simulink library "aero"  (R2022b)
settings: Solver=VariableStepAuto  StartTime=0.0  StopTime=10.0  RelTol=1e-3
values from neighbouring files (symbols this model uses):
  alpha_da = (-3:3:12)'    [load_mdl_data.m]
  alpha_de = (-2:2:14)'    [load_mdl_data.m]
  alpha_dr = (-3:3:12)'    [load_mdl_data.m]
  alpha_dyn = [4,6,8]    [load_mdl_data.m]
  alpha_lat = (-2:2:8)'    [load_mdl_data.m]
  alpha_lon = (-2:2:18)'    [load_mdl_data.m]
  beta_lat = -6:3:6    [load_mdl_data.m]
  CD_base = data_base(:,2)    [load_mdl_data.m]
  CD_beta = [data_beta_n6(:,2)-interp1(alpha_lon,CD_base, alpha_lat),      data_beta_n3(:,2)-interp1(alpha_lon,CD_base, alpha_lat),      zeros(size(data_beta_n3(:,2))),      data_beta_p3(:,2)-interp1(alpha_lon,CD_base, alpha_lat),      data_beta_p6(:,2)-interp1(alpha_lon,CD_base, alpha_lat)]    [load_mdl_data.m]
  CD_da = [data_da_n15(:,2)-interp1(alpha_lon,CD_base, alpha_da,'linear','extrap'),      zeros(size(data_da_n15(:,2))),      data_da_p15(:,2)-interp1(alpha_lon,CD_base, alpha_da,'linear','extrap')]/15    [load_mdl_data.m]
  CD_de = [(data_de_n15(:,2)-interp1(alpha_lon,CD_base, alpha_de,'linear','extrap'))/-15,      (data_de_p15(:,2)-data_de_n15(:,2))/30,      (data_de_p15(:,2)-interp1(alpha_lon,CD_base, alpha_de,'linear','extrap'))/15]    [load_mdl_data.m]
  CD_dr = [data_dr_n15(:,2)-interp1(alpha_lon,CD_base, alpha_dr,'linear','extrap'),      zeros(size(data_dr_n15(:,2))),      data_dr_p15(:,2)-interp1(alpha_lon,CD_base, alpha_dr,'linear','extrap')]/15    [load_mdl_data.m]
  CL_base = data_base(:,1)    [load_mdl_data.m]
  Cl_base = data_base(:,5)    [load_mdl_data.m]
  CL_beta = [data_beta_n6(:,1)-interp1(alpha_lon,CL_base, alpha_lat),      data_beta_n3(:,1)-interp1(alpha_lon,CL_base, alpha_lat),      zeros(size(data_beta_n3(:,1))),      data_beta_p3(:,1)-interp1(alpha_lon,CL_base, alpha_lat),      data_beta_p6(:,1)-interp1(alpha_lon,CL_base, alpha_lat)]    [load_mdl_data.m]
  Cl_beta = [data_beta_n6(:,5)-interp1(alpha_lon,Cl_base, alpha_lat),      data_beta_n3(:,5)-interp1(alpha_lon,Cl_base, alpha_lat),      zeros(size(data_beta_n3(:,5))),      data_beta_p3(:,5)-interp1(alpha_lon,Cl_base, alpha_lat),      data_beta_p6(:,5)-interp1(alpha_lon,Cl_base, alpha_lat)]    [load_mdl_data.m]
  CL_da = [data_da_n15(:,1)-interp1(alpha_lon,CL_base, alpha_da,'linear','extrap'),      zeros(size(data_da_n15(:,1))),      data_da_p15(:,1)-interp1(alpha_lon,CL_base, alpha_da,'linear','extrap')]/15    [load_mdl_data.m]
  Cl_da = [(data_da_n15(:,5)-interp1(alpha_lon,Cl_base, alpha_da,'linear','extrap'))/-15,      (data_da_p15(:,5)-data_da_n15(:,5))/30,      (data_da_p15(:,5)-interp1(alpha_lon,Cl_base, alpha_da,'linear','extrap'))/15]    [load_mdl_data.m]
  CL_de = [(data_de_n15(:,1)-interp1(alpha_lon,CL_base, alpha_de,'linear','extrap'))/-15,      (data_de_p15(:,1)-data_de_n15(:,1))/30,      (data_de_p15(:,1)-interp1(alpha_lon,CL_base, alpha_de,'linear','extrap'))/15]    [load_mdl_data.m]
  CL_dr = [data_dr_n15(:,1)-interp1(alpha_lon,CL_base, alpha_dr,'linear','extrap'),      zeros(size(data_dr_n15(:,1))),      data_dr_p15(:,1)-interp1(alpha_lon,CL_base, alpha_dr,'linear','extrap')]/15    [load_mdl_data.m]
  Cl_dr = [(data_dr_n15(:,5)-interp1(alpha_lon,Cl_base, alpha_dr,'linear','extrap'))/-15,      (data_dr_p15(:,5)-data_dr_n15(:,5))/30,      (data_dr_p15(:,5)-interp1(alpha_lon,Cl_base, alpha_dr,'linear','extrap'))/15]    [load_mdl_data.m]
  Clp = [-0.7,  -0.66, -0.58]    [load_mdl_data.m]
  CLq = [71,    60,    55]    [load_mdl_data.m]
  Clr = [0.39,   0.45,  0.52]    [load_mdl_data.m]
  Cm_base = data_base(:,4)    [load_mdl_data.m]
  Cm_beta = [data_beta_n6(:,4)-interp1(alpha_lon,Cm_base, alpha_lat),      data_beta_n3(:,4)-interp1(alpha_lon,Cm_base, alpha_lat),      zeros(size(data_beta_n3(:,4))),      data_beta_p3(:,4)-interp1(alpha_lon,Cm_base, alpha_lat),      data_beta_p6(:,4)-interp1(alpha_lon,Cm_base, alpha_lat)]    [load_mdl_data.m]
  Cm_da = [data_da_n15(:,4)-interp1(alpha_lon,Cm_base, alpha_da,'linear','extrap'),      zeros(size(data_da_n15(:,4))),      data_da_p15(:,4)-interp1(alpha_lon,Cm_base, alpha_da,'linear','extrap')]/15    [load_mdl_data.m]
  Cm_de = [(data_de_n15(:,4)-interp1(alpha_lon,Cm_base, alpha_de,'linear','extrap'))/-15,      (data_de_p15(:,4)-data_de_n15(:,4))/30,      (data_de_p15(:,4)-interp1(alpha_lon,Cm_base, alpha_de,'linear','extrap'))/15]    [load_mdl_data.m]
  Cm_dr = [data_dr_n15(:,4)-interp1(alpha_lon,Cm_base, alpha_dr,'linear','extrap'),      zeros(size(data_dr_n15(:,4))),      data_dr_p15(:,4)-interp1(alpha_lon,Cm_base, alpha_dr,'linear','extrap')]/15    [load_mdl_data.m]
  Cmq = [-54,  -55,   -55]    [load_mdl_data.m]
  Cn_base = data_base(:,6)    [load_mdl_data.m]
  Cn_beta = [data_beta_n6(:,6)-interp1(alpha_lon,Cn_base, alpha_lat),      data_beta_n3(:,6)-interp1(alpha_lon,Cn_base, alpha_lat),      zeros(size(data_beta_n3(:,6))),      data_beta_p3(:,6)-interp1(alpha_lon,Cn_base, alpha_lat),      data_beta_p6(:,6)-interp1(alpha_lon,Cn_base, alpha_lat)]    [load_mdl_data.m]
  Cn_da = [(data_da_n15(:,6)-interp1(alpha_lon,Cn_base, alpha_da,'linear','extrap'))/-15,      (data_da_p15(:,6)-data_da_n15(:,6))/30,      (data_da_p15(:,6)-interp1(alpha_lon,Cn_base, alpha_da,'linear','extrap'))/15]    [load_mdl_data.m]
  Cn_dr = [(data_dr_n15(:,6)-interp1(alpha_lon,Cn_base, alpha_dr,'linear','extrap'))/-15,      (data_dr_p15(:,6)-data_dr_n15(:,6))/30,      (data_dr_p15(:,6)-interp1(alpha_lon,Cn_base, alpha_dr,'linear','extrap'))/15]    [load_mdl_data.m]
  Cnp = [-0.07, -0.08, -0.09]    [load_mdl_data.m]
  Cnr = [-0.12, -0.13, -0.14]    [load_mdl_data.m]
  Cs_base = data_base(:,3)    [load_mdl_data.m]
  Cs_beta = [data_beta_n6(:,3)-interp1(alpha_lon,Cs_base, alpha_lat),      data_beta_n3(:,3)-interp1(alpha_lon,Cs_base, alpha_lat),      zeros(size(data_beta_n3(:,3))),      data_beta_p3(:,3)-interp1(alpha_lon,Cs_base, alpha_lat),      data_beta_p6(:,3)-interp1(alpha_lon,Cs_base, alpha_lat)]    [load_mdl_data.m]
  Cs_da = [(data_da_n15(:,3)-interp1(alpha_lon,Cs_base, alpha_da,'linear','extrap'))/-15,      (data_da_p15(:,3)-data_da_n15(:,3))/30,      (data_da_p15(:,3)-interp1(alpha_lon,Cs_base, alpha_da,'linear','extrap'))/15]    [load_mdl_data.m]
  Cs_dr = [(data_dr_n15(:,3)-interp1(alpha_lon,Cs_base, alpha_dr,'linear','extrap'))/-15,      (data_dr_p15(:,3)-data_dr_n15(:,3))/30,      (data_dr_p15(:,3)-interp1(alpha_lon,Cs_base, alpha_dr,'linear','extrap'))/15]    [load_mdl_data.m]
  da_bp = [-15 0 15]    [load_mdl_data.m]
  de_bp = [-15 0 15]    [load_mdl_data.m]
  dr_bp = [-15 0 15]    [load_mdl_data.m]
  RefLen = 0.18    [load_mdl_data.m]
  RefSpan = 3.2    [load_mdl_data.m]
libraries: simulink_extras x5
settings Model: Creator=matt  LastModifiedBy=matt

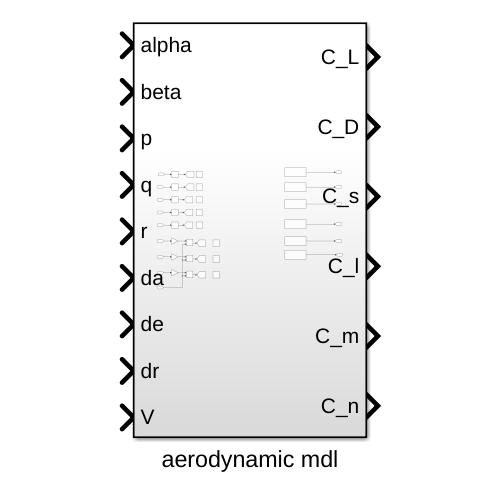
[thumbnail: Simulink's stored preview of the top-level diagram]
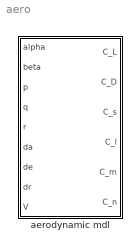
== system aero ==
  aerodynamic mdl : Subsystem

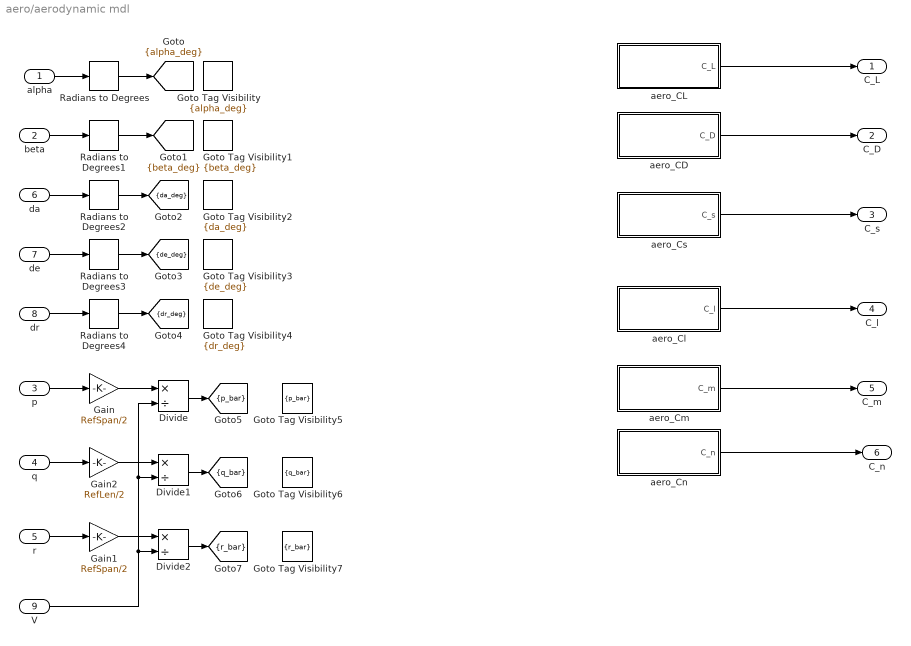
== system aero/aerodynamic mdl ==
  alpha : Inport
  beta : Inport  Port=2
  p : Inport  Port=3
  q : Inport  Port=4
  r : Inport  Port=5
  da : Inport  Port=6
  de : Inport  Port=7
  dr : Inport  Port=8
  V : Inport  Port=9
  Divide : Product  Inputs=*/
  Divide1 : Product  Inputs=*/
  Divide2 : Product  Inputs=*/
  Gain : Gain  Gain=RefSpan/2
  Gain1 : Gain  Gain=RefSpan/2
  Gain2 : Gain  Gain=RefLen/2
  Goto Tag Visibility : GotoTagVisibility  GotoTag=alpha_deg
  Goto Tag Visibility1 : GotoTagVisibility  GotoTag=beta_deg
  Goto Tag Visibility2 : GotoTagVisibility  GotoTag=da_deg
  Goto Tag Visibility3 : GotoTagVisibility  GotoTag=de_deg
  Goto Tag Visibility4 : GotoTagVisibility  GotoTag=dr_deg
  Goto Tag Visibility5 : GotoTagVisibility  GotoTag=p_bar
  Goto Tag Visibility6 : GotoTagVisibility  GotoTag=q_bar
  Goto Tag Visibility7 : GotoTagVisibility  GotoTag=r_bar
  Radians to Degrees{,1..4} (5 alike) : simulink_extras/Transformations/Radians to Degrees
  aero_CD : Subsystem
  aero_CL : Subsystem
  aero_Cl : Subsystem
  aero_Cm : Subsystem
  aero_Cn : Subsystem
  aero_Cs : Subsystem
  C_L : Outport
  C_D : Outport  Port=2
  C_s : Outport  Port=3
  C_l : Outport  Port=4
  C_m : Outport  Port=5
  C_n : Outport  Port=6
  tag scope: alpha_deg=scoped, beta_deg=scoped, da_deg=scoped, de_deg=scoped, dr_deg=scoped, p_bar=scoped, q_bar=scoped, r_bar=scoped
  wires:
  alpha/1 -> Radians to Degrees/1
  beta/1 -> Radians to Degrees1/1
  Radians to Degrees/1 -> [alpha_deg]
  Radians to Degrees1/1 -> [beta_deg]
  dr/1 -> Radians to Degrees4/1
  de/1 -> Radians to Degrees3/1
  da/1 -> Radians to Degrees2/1
  Radians to Degrees2/1 -> [da_deg]
  Radians to Degrees3/1 -> [de_deg]
  Radians to Degrees4/1 -> [dr_deg]
  p/1 -> Gain/1
  r/1 -> Gain1/1
  q/1 -> Gain2/1
  Gain/1 -> Divide/1
  V/1 -> Divide2/2, Divide1/2, Divide/2
  Divide/1 -> [p_bar]
  Divide1/1 -> [q_bar]
  Gain2/1 -> Divide1/1
  Divide2/1 -> [r_bar]
  Gain1/1 -> Divide2/1
  aero_CL/1(C_L) -> C_L/1
  aero_Cm/1(C_m) -> C_m/1
  aero_CD/1(C_D) -> C_D/1
  aero_Cs/1(C_s) -> C_s/1
  aero_Cl/1(C_l) -> C_l/1
  aero_Cn/1(C_n) -> C_n/1

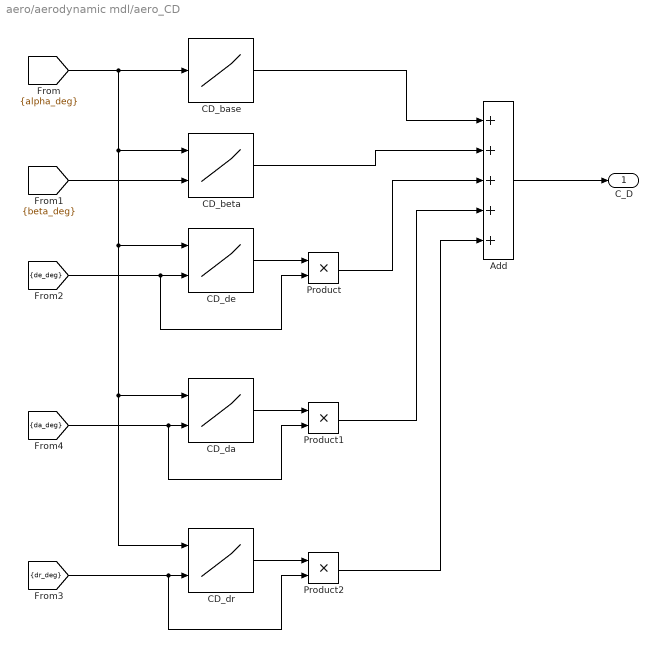
== system aero/aerodynamic mdl/aero_CD ==
  Add : Sum  Inputs=+++++
  CD_base : Lookup_n-D  NumberOfTableDimensions=1  BreakpointsForDimension1=alpha_lon  BeginIndexSearchUsingPreviousIndexResult=on  Table=CD_base  InternalRulePriority=Speed  RndMeth=Simplest
  CD_beta : Lookup_n-D  BreakpointsForDimension1=alpha_lat  BreakpointsForDimension2=beta_lat  BeginIndexSearchUsingPreviousIndexResult=on  Table=CD_beta  InternalRulePriority=Speed  RndMeth=Simplest
      settings: InputPortMap=u0,u1
  CD_da : Lookup_n-D  BreakpointsForDimension1=alpha_da  BreakpointsForDimension2=da_bp  BeginIndexSearchUsingPreviousIndexResult=on  Table=CD_da  ExtrapMethod=Clip  InternalRulePriority=Speed  RndMeth=Simplest
      settings: InputPortMap=u0,u1
  CD_de : Lookup_n-D  BreakpointsForDimension1=alpha_de  BreakpointsForDimension2=de_bp  BeginIndexSearchUsingPreviousIndexResult=on  Table=CD_de  ExtrapMethod=Clip  InternalRulePriority=Speed  RndMeth=Simplest
      settings: InputPortMap=u0,u1
  CD_dr : Lookup_n-D  BreakpointsForDimension1=alpha_dr  BreakpointsForDimension2=dr_bp  BeginIndexSearchUsingPreviousIndexResult=on  Table=CD_dr  ExtrapMethod=Clip  InternalRulePriority=Speed  RndMeth=Simplest
      settings: InputPortMap=u0,u1
  Product : Product
  Product1 : Product
  Product2 : Product
  C_D : Outport
  wires:
  Product2/1 -> Add/5
  [dr_deg] -> CD_dr/2, Product2/2
  CD_dr/1 -> Product2/1
  [alpha_deg] -> CD_base/1, CD_beta/1, CD_de/1, CD_da/1, CD_dr/1
  Product1/1 -> Add/4
  [da_deg] -> CD_da/2, Product1/2
  CD_da/1 -> Product1/1
  Product/1 -> Add/3
  [de_deg] -> CD_de/2, Product/2
  CD_de/1 -> Product/1
  [beta_deg] -> CD_beta/2
  CD_beta/1 -> Add/2
  CD_base/1 -> Add/1
  Add/1 -> C_D/1

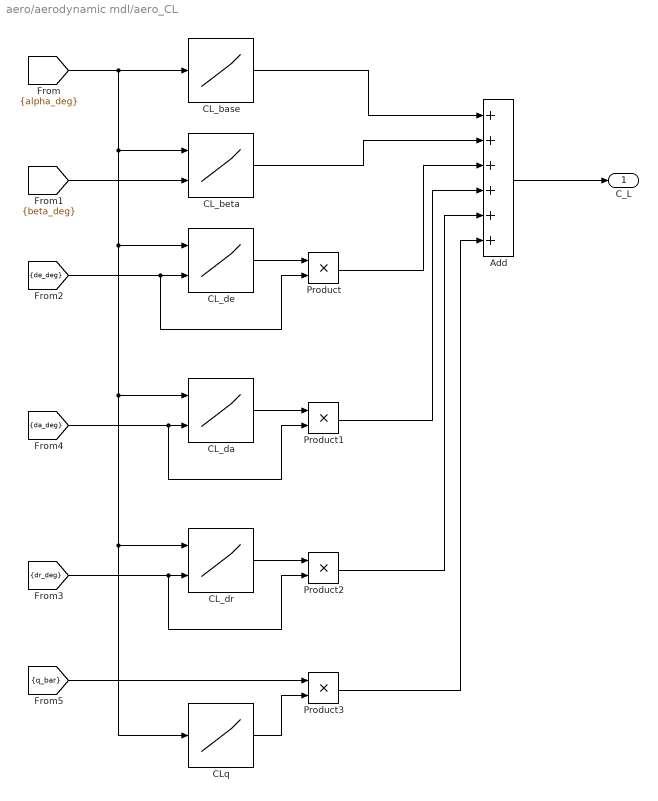
== system aero/aerodynamic mdl/aero_CL ==
  Add : Sum  Inputs=++++++
  CL_base : Lookup_n-D  NumberOfTableDimensions=1  BreakpointsForDimension1=alpha_lon  BeginIndexSearchUsingPreviousIndexResult=on  Table=CL_base  InternalRulePriority=Speed  RndMeth=Simplest
  CL_beta : Lookup_n-D  BreakpointsForDimension1=alpha_lat  BreakpointsForDimension2=beta_lat  BeginIndexSearchUsingPreviousIndexResult=on  Table=CL_beta  InternalRulePriority=Speed  RndMeth=Simplest
      settings: InputPortMap=u0,u1
  CL_da : Lookup_n-D  BreakpointsForDimension1=alpha_da  BreakpointsForDimension2=da_bp  BeginIndexSearchUsingPreviousIndexResult=on  Table=CL_da  ExtrapMethod=Clip  InternalRulePriority=Speed  RndMeth=Simplest
      settings: InputPortMap=u0,u1
  CL_de : Lookup_n-D  BreakpointsForDimension1=alpha_de  BreakpointsForDimension2=de_bp  BeginIndexSearchUsingPreviousIndexResult=on  Table=CL_de  ExtrapMethod=Clip  InternalRulePriority=Speed  RndMeth=Simplest
      settings: InputPortMap=u0,u1
  CL_dr : Lookup_n-D  BreakpointsForDimension1=alpha_dr  BreakpointsForDimension2=dr_bp  BeginIndexSearchUsingPreviousIndexResult=on  Table=CL_dr  ExtrapMethod=Clip  InternalRulePriority=Speed  RndMeth=Simplest
      settings: InputPortMap=u0,u1
  CLq : Lookup_n-D  NumberOfTableDimensions=1  BreakpointsForDimension1=alpha_dyn  BeginIndexSearchUsingPreviousIndexResult=on  Table=CLq  ExtrapMethod=Clip  UseLastTableValue=on  InternalRulePriority=Speed  RndMeth=Simplest
  Product{,1..3} (4 alike) : Product
  C_L : Outport
  wires:
  Add/1 -> C_L/1
  CL_base/1 -> Add/1
  CL_beta/1 -> Add/2
  [beta_deg] -> CL_beta/2
  CL_de/1 -> Product/1
  [de_deg] -> Product/2, CL_de/2
  Product/1 -> Add/3
  CL_da/1 -> Product1/1
  [da_deg] -> Product1/2, CL_da/2
  Product1/1 -> Add/4
  [alpha_deg] -> CLq/1, CL_dr/1, CL_da/1, CL_de/1, CL_beta/1, CL_base/1
  CL_dr/1 -> Product2/1
  [dr_deg] -> Product2/2, CL_dr/2
  Product2/1 -> Add/5
  [q_bar] -> Product3/1
  Product3/1 -> Add/6
  CLq/1 -> Product3/2

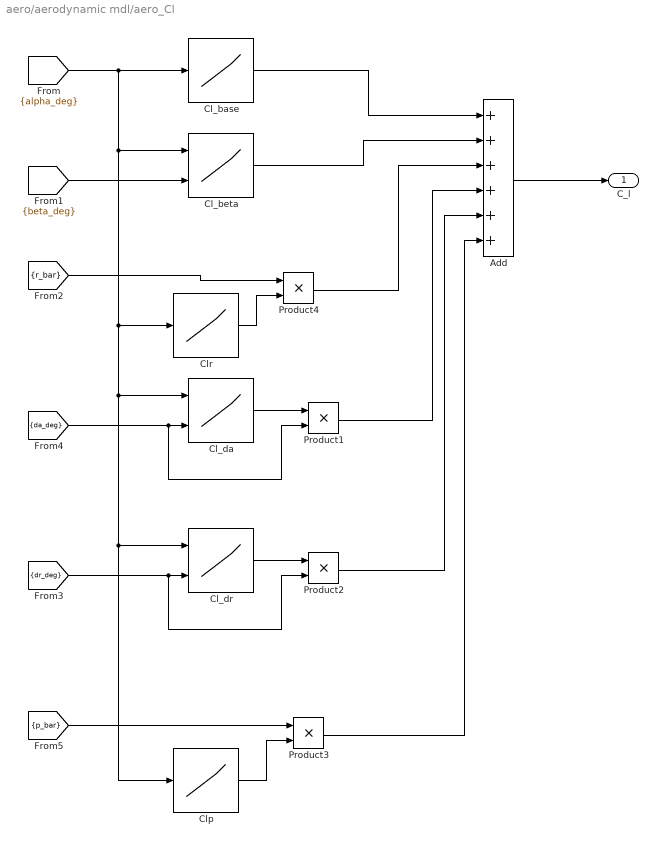
== system aero/aerodynamic mdl/aero_Cl ==
  Add : Sum  Inputs=++++++
  Cl_base : Lookup_n-D  NumberOfTableDimensions=1  BreakpointsForDimension1=alpha_lon  BeginIndexSearchUsingPreviousIndexResult=on  Table=Cl_base  InternalRulePriority=Speed  RndMeth=Simplest
  Cl_beta : Lookup_n-D  BreakpointsForDimension1=alpha_lat  BreakpointsForDimension2=beta_lat  BeginIndexSearchUsingPreviousIndexResult=on  Table=Cl_beta  InternalRulePriority=Speed  RndMeth=Simplest
      settings: InputPortMap=u0,u1
  Cl_da : Lookup_n-D  BreakpointsForDimension1=alpha_da  BreakpointsForDimension2=da_bp  BeginIndexSearchUsingPreviousIndexResult=on  Table=Cl_da  ExtrapMethod=Clip  InternalRulePriority=Speed  RndMeth=Simplest
      settings: InputPortMap=u0,u1
  Cl_dr : Lookup_n-D  BreakpointsForDimension1=alpha_dr  BreakpointsForDimension2=dr_bp  BeginIndexSearchUsingPreviousIndexResult=on  Table=Cl_dr  ExtrapMethod=Clip  InternalRulePriority=Speed  RndMeth=Simplest
      settings: InputPortMap=u0,u1
  Clp : Lookup_n-D  NumberOfTableDimensions=1  BreakpointsForDimension1=alpha_dyn  BeginIndexSearchUsingPreviousIndexResult=on  Table=Clp  ExtrapMethod=Clip  UseLastTableValue=on  InternalRulePriority=Speed  RndMeth=Simplest
  Clr : Lookup_n-D  NumberOfTableDimensions=1  BreakpointsForDimension1=alpha_dyn  BeginIndexSearchUsingPreviousIndexResult=on  Table=Clr  ExtrapMethod=Clip  UseLastTableValue=on  InternalRulePriority=Speed  RndMeth=Simplest
  Product{1..4} (4 alike) : Product
  C_l : Outport
  wires:
  Add/1 -> C_l/1
  Cl_base/1 -> Add/1
  Cl_beta/1 -> Add/2
  [beta_deg] -> Cl_beta/2
  Cl_da/1 -> Product1/1
  [da_deg] -> Product1/2, Cl_da/2
  Product1/1 -> Add/4
  [alpha_deg] -> Clp/1, Cl_dr/1, Cl_da/1, Clr/1, Cl_beta/1, Cl_base/1
  Cl_dr/1 -> Product2/1
  [dr_deg] -> Product2/2, Cl_dr/2
  Product2/1 -> Add/5
  [p_bar] -> Product3/1
  Product3/1 -> Add/6
  [r_bar] -> Product4/1
  Product4/1 -> Add/3
  Clp/1 -> Product3/2
  Clr/1 -> Product4/2

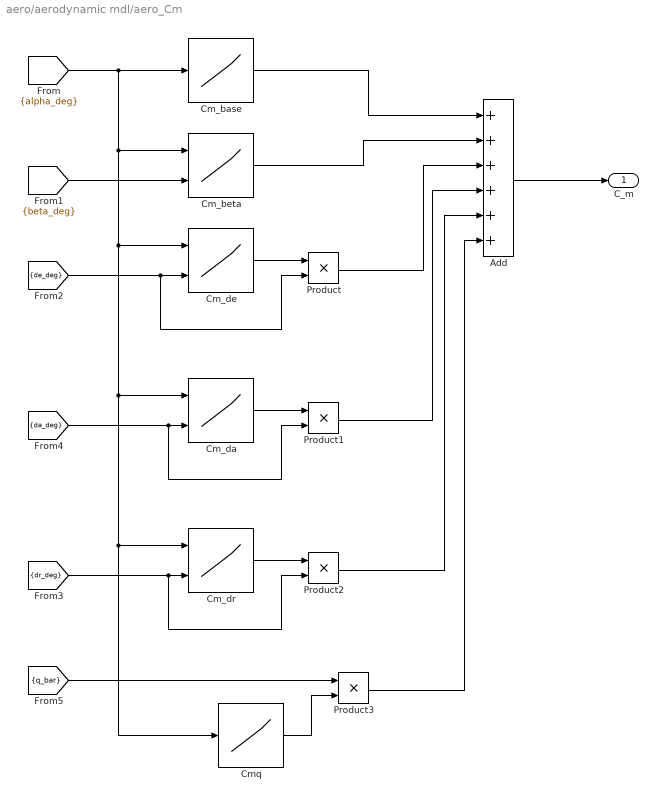
== system aero/aerodynamic mdl/aero_Cm ==
  Add : Sum  Inputs=++++++
  Cm_base : Lookup_n-D  NumberOfTableDimensions=1  BreakpointsForDimension1=alpha_lon  BeginIndexSearchUsingPreviousIndexResult=on  Table=Cm_base  InternalRulePriority=Speed  RndMeth=Simplest
  Cm_beta : Lookup_n-D  BreakpointsForDimension1=alpha_lat  BreakpointsForDimension2=beta_lat  BeginIndexSearchUsingPreviousIndexResult=on  Table=Cm_beta  InternalRulePriority=Speed  RndMeth=Simplest
      settings: InputPortMap=u0,u1
  Cm_da : Lookup_n-D  BreakpointsForDimension1=alpha_da  BreakpointsForDimension2=da_bp  BeginIndexSearchUsingPreviousIndexResult=on  Table=Cm_da  ExtrapMethod=Clip  InternalRulePriority=Speed  RndMeth=Simplest
      settings: InputPortMap=u0,u1
  Cm_de : Lookup_n-D  BreakpointsForDimension1=alpha_de  BreakpointsForDimension2=de_bp  BeginIndexSearchUsingPreviousIndexResult=on  Table=Cm_de  ExtrapMethod=Clip  InternalRulePriority=Speed  RndMeth=Simplest
      settings: InputPortMap=u0,u1
  Cm_dr : Lookup_n-D  BreakpointsForDimension1=alpha_dr  BreakpointsForDimension2=dr_bp  BeginIndexSearchUsingPreviousIndexResult=on  Table=Cm_dr  ExtrapMethod=Clip  InternalRulePriority=Speed  RndMeth=Simplest
      settings: InputPortMap=u0,u1
  Cmq : Lookup_n-D  NumberOfTableDimensions=1  BreakpointsForDimension1=alpha_dyn  BeginIndexSearchUsingPreviousIndexResult=on  Table=Cmq  ExtrapMethod=Clip  UseLastTableValue=on  InternalRulePriority=Speed  RndMeth=Simplest
  Product{,1..3} (4 alike) : Product
  C_m : Outport
  wires:
  Product3/1 -> Add/6
  [q_bar] -> Product3/1
  Product2/1 -> Add/5
  [dr_deg] -> Cm_dr/2, Product2/2
  Cm_dr/1 -> Product2/1
  [alpha_deg] -> Cm_base/1, Cm_beta/1, Cm_de/1, Cm_da/1, Cmq/1, Cm_dr/1
  Product1/1 -> Add/4
  [da_deg] -> Cm_da/2, Product1/2
  Cm_da/1 -> Product1/1
  Product/1 -> Add/3
  [de_deg] -> Cm_de/2, Product/2
  Cm_de/1 -> Product/1
  [beta_deg] -> Cm_beta/2
  Cm_beta/1 -> Add/2
  Cm_base/1 -> Add/1
  Add/1 -> C_m/1
  Cmq/1 -> Product3/2

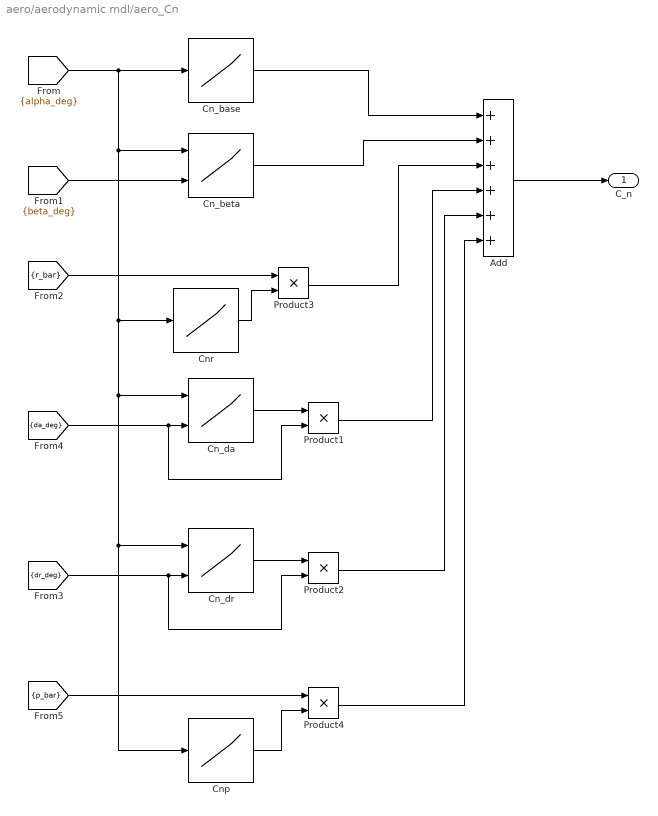
== system aero/aerodynamic mdl/aero_Cn ==
  Add : Sum  Inputs=++++++
  Cn_base : Lookup_n-D  NumberOfTableDimensions=1  BreakpointsForDimension1=alpha_lon  BeginIndexSearchUsingPreviousIndexResult=on  Table=Cn_base  InternalRulePriority=Speed  RndMeth=Simplest
  Cn_beta : Lookup_n-D  BreakpointsForDimension1=alpha_lat  BreakpointsForDimension2=beta_lat  BeginIndexSearchUsingPreviousIndexResult=on  Table=Cn_beta  InternalRulePriority=Speed  RndMeth=Simplest
      settings: InputPortMap=u0,u1
  Cn_da : Lookup_n-D  BreakpointsForDimension1=alpha_da  BreakpointsForDimension2=da_bp  BeginIndexSearchUsingPreviousIndexResult=on  Table=Cn_da  ExtrapMethod=Clip  InternalRulePriority=Speed  RndMeth=Simplest
      settings: InputPortMap=u0,u1
  Cn_dr : Lookup_n-D  BreakpointsForDimension1=alpha_dr  BreakpointsForDimension2=dr_bp  BeginIndexSearchUsingPreviousIndexResult=on  Table=Cn_dr  ExtrapMethod=Clip  InternalRulePriority=Speed  RndMeth=Simplest
      settings: InputPortMap=u0,u1
  Cnp : Lookup_n-D  NumberOfTableDimensions=1  BreakpointsForDimension1=alpha_dyn  BeginIndexSearchUsingPreviousIndexResult=on  Table=Cnp  ExtrapMethod=Clip  UseLastTableValue=on  InternalRulePriority=Speed  RndMeth=Simplest
  Cnr : Lookup_n-D  NumberOfTableDimensions=1  BreakpointsForDimension1=alpha_dyn  BeginIndexSearchUsingPreviousIndexResult=on  Table=Cnr  ExtrapMethod=Clip  UseLastTableValue=on  InternalRulePriority=Speed  RndMeth=Simplest
  Product{1..4} (4 alike) : Product
  C_n : Outport
  wires:
  Add/1 -> C_n/1
  Cn_base/1 -> Add/1
  Cn_beta/1 -> Add/2
  [beta_deg] -> Cn_beta/2
  Cn_da/1 -> Product1/1
  [da_deg] -> Product1/2, Cn_da/2
  Product1/1 -> Add/4
  [alpha_deg] -> Cnp/1, Cn_dr/1, Cn_da/1, Cnr/1, Cn_beta/1, Cn_base/1
  Cn_dr/1 -> Product2/1
  [dr_deg] -> Product2/2, Cn_dr/2
  Product2/1 -> Add/5
  [p_bar] -> Product4/1
  Product4/1 -> Add/6
  [r_bar] -> Product3/1
  Product3/1 -> Add/3
  Cnr/1 -> Product3/2
  Cnp/1 -> Product4/2

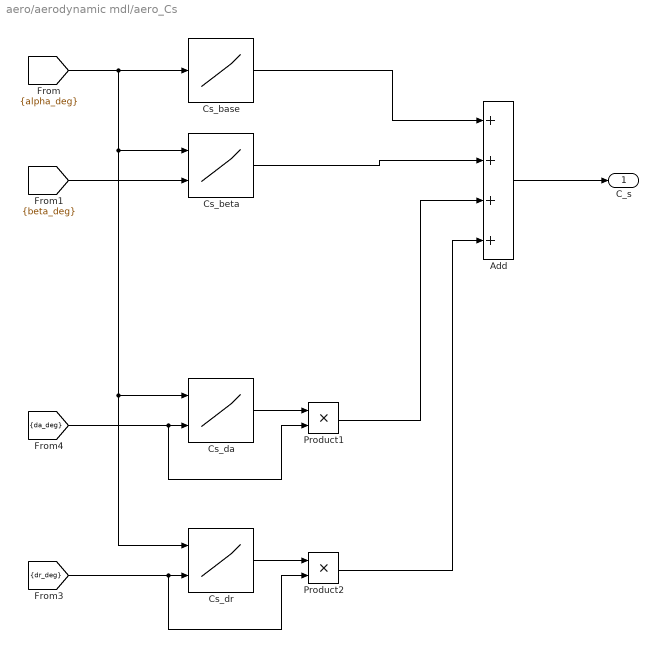
== system aero/aerodynamic mdl/aero_Cs ==
  Add : Sum  Inputs=++++
  Cs_base : Lookup_n-D  NumberOfTableDimensions=1  BreakpointsForDimension1=alpha_lon  BeginIndexSearchUsingPreviousIndexResult=on  Table=Cs_base  InternalRulePriority=Speed  RndMeth=Simplest
  Cs_beta : Lookup_n-D  BreakpointsForDimension1=alpha_lat  BreakpointsForDimension2=beta_lat  BeginIndexSearchUsingPreviousIndexResult=on  Table=Cs_beta  InternalRulePriority=Speed  RndMeth=Simplest
      settings: InputPortMap=u0,u1
  Cs_da : Lookup_n-D  BreakpointsForDimension1=alpha_da  BreakpointsForDimension2=da_bp  BeginIndexSearchUsingPreviousIndexResult=on  Table=Cs_da  ExtrapMethod=Clip  InternalRulePriority=Speed  RndMeth=Simplest
      settings: InputPortMap=u0,u1
  Cs_dr : Lookup_n-D  BreakpointsForDimension1=alpha_dr  BreakpointsForDimension2=dr_bp  BeginIndexSearchUsingPreviousIndexResult=on  Table=Cs_dr  ExtrapMethod=Clip  InternalRulePriority=Speed  RndMeth=Simplest
      settings: InputPortMap=u0,u1
  Product1 : Product
  Product2 : Product
  C_s : Outport
  wires:
  Add/1 -> C_s/1
  Cs_base/1 -> Add/1
  Cs_beta/1 -> Add/2
  [beta_deg] -> Cs_beta/2
  Cs_da/1 -> Product1/1
  [da_deg] -> Product1/2, Cs_da/2
  Product1/1 -> Add/3
  [alpha_deg] -> Cs_dr/1, Cs_da/1, Cs_beta/1, Cs_base/1
  Cs_dr/1 -> Product2/1
  [dr_deg] -> Product2/2, Cs_dr/2
  Product2/1 -> Add/4
